simulink library "dit"  (Simulink 8.1)
settings: Solver=ode1  StartTime=0.0  StopTime=Inf  FixedStep=0.001  RelTol=1e-3
PostLoadFcn:
  | , if any(exist('dsrtsu_mdlpostloadfcn', 'file') == [2, 3, 6]), try dsrtsu_mdlpostloadfcn('Execute', bdroot); catch fprintf('Error in PostLoadFcn (dsrtsu_mdlpostloadfcn) for model "%s":\n %s\n', bdroot, lasterr); end, end,
undefined symbols (not defined in the file or in its folder): KACC_TransDistIncMargin_m, KACC_TransitoryClearanceDec_m, KACC_TransitoryDesDistApproach_m, KACC_TransitoryDistIntrusion_m, KACC_TransitoryRelSpd_kph
libraries: hcu_lib x1
settings Model: DSRTSU_INTERNAL_RTI_VER=450  DSRTSU_INTERNAL_RTI_TYPE=rti1401  RTICANMMDATA=struct('GeneralSetupData',struct('modelroot','D:\ELN150201_TAIWAN\trunk\AdasDragon\software\sw_development\arch\app\acc','generalsettings',struct('filesettings',struct('destfolder',struct('Name','RTICANMM_FILES','Check',1),'buildfolder',struct('Name','.','Check',1),'AbsDestfolder',struct('Name','D:\ELN150201_TAIWAN\trunk\AdasDragon\software\sw_development\arch\app\acc\RTICANMM_FILES'),'AbsBuildfolder',struct('Name','D:\ELN150201_TAIWAN\trunk\AdasDragon\software\sw_development\arch\app\acc'))),'options',struct('addpaths',1,'rmpaths',1,'addtrcexclusion',logical(1),'cannavigator',struct('checkmonitoring',0),'show_usrtrc',0,'use_usrtrc',0),'advanced',struct('options',[1 1 1 1 1 1 1 1 1 1 1 1 1 1 1 1 1 1 1 1 1 1 1 1 1 1 1 1 1 1 1 1 1 1 1 1 1 1 1 1 1 1 1 1 1 1 1 1 1 1 1 1 1 1 1 1 1 1 1 1 1 1 1 1 1 1 1 1 1 1 1 1 1 1 1 1 1 1 1 1 1 1 1 1 1 1 1 1 1 1 1 1 1 1 1 1 1 1 1 1]),'MPSetup',{{}},'modelname','dit','block','dit'))  DSRTSU_INTERNAL_RTIFPGA=40  Creator=AT015411  LastModifiedBy=AT015555

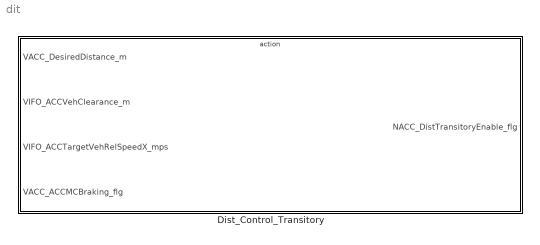
== system dit ==
  Dist_Control_Transitory : Subsystem  TreatAsAtomicUnit=on

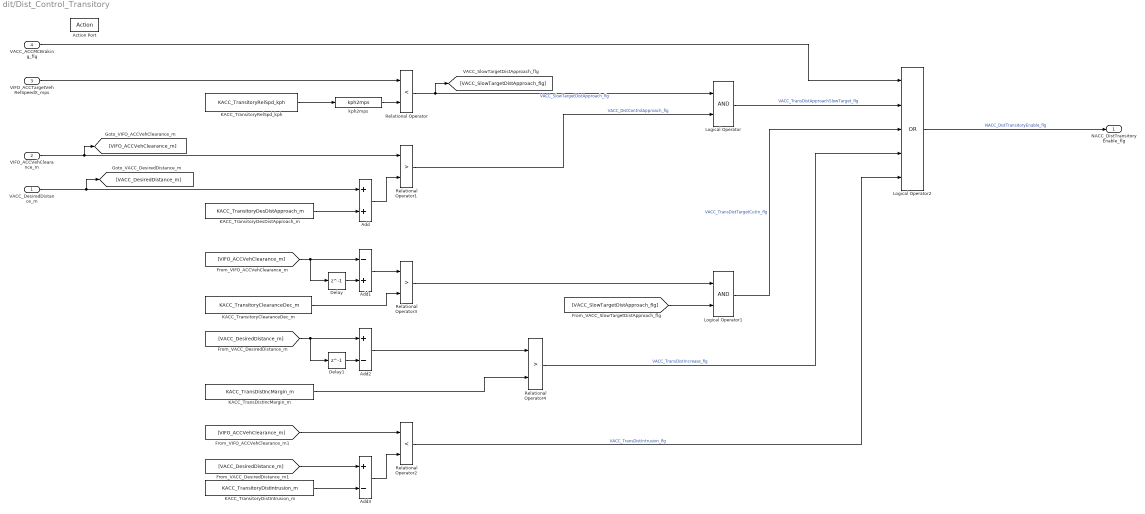
== system dit/Dist_Control_Transitory ==
  VACC_DesiredDistance_m : Inport
  VIFO_ACCVehClearance_m : Inport  Port=2
  VIFO_ACCTargetVehRelSpeedX_mps : Inport  Port=3
  VACC_ACCMCBraking_flg : Inport  Port=4
  Action Port : ActionPort
  Add : Sum
  Add1 : Sum  Inputs=-+
  Add2 : Sum  Inputs=+-
  Add3 : Sum  Inputs=+-
  Delay : Delay  DelayLength=1  InitialCondition=0
  Delay1 : Delay  DelayLength=1  InitialCondition=0
  KACC_TransDistIncMargin_m : Constant  Value=KACC_TransDistIncMargin_m
  KACC_TransitoryClearanceDec_m : Constant  Value=KACC_TransitoryClearanceDec_m
  KACC_TransitoryDesDistApproach_m : Constant  Value=KACC_TransitoryDesDistApproach_m
  KACC_TransitoryDistIntrusion_m : Constant  Value=KACC_TransitoryDistIntrusion_m
  KACC_TransitoryRelSpd_kph : Constant  Value=KACC_TransitoryRelSpd_kph
  Logical Operator : Logic  AllPortsSameDT=off  OutDataTypeStr=boolean
  Logical Operator1 : Logic  AllPortsSameDT=off  OutDataTypeStr=boolean
  Logical Operator2 : Logic  Operator=OR  Inputs=5  AllPortsSameDT=off  OutDataTypeStr=boolean
  Relational Operator : RelationalOperator  Operator=<  OutDataTypeStr=boolean
  Relational Operator1 : RelationalOperator  Operator=>  OutDataTypeStr=boolean
  Relational Operator2 : RelationalOperator  Operator=<  OutDataTypeStr=boolean
  Relational Operator3 : RelationalOperator  Operator=>  OutDataTypeStr=boolean
  Relational Operator4 : RelationalOperator  Operator=>  OutDataTypeStr=boolean
  kph2mps : hcu_lib/kph2mps
  NACC_DistTransitoryEnable_flg : Outport
  wires:
  VIFO_ACCTargetVehRelSpeedX_mps/1 -> Relational Operator/1
  KACC_TransitoryRelSpd_kph/1 -> kph2mps/1
  kph2mps/1 -> Relational Operator/2
  VIFO_ACCVehClearance_m/1 -> [VIFO_ACCVehClearance_m], Relational Operator1/1
  VACC_DesiredDistance_m/1 -> [VACC_DesiredDistance_m], Add/1
  KACC_TransitoryDesDistApproach_m/1 -> Add/2
  Add/1 -> Relational Operator1/2
  Relational Operator/1 -> Logical Operator/1, [VACC_SlowTargetDistApproach_flg]  "VACC_SlowTargetDistApproach_flg"
  Relational Operator1/1 -> Logical Operator/2  "VACC_DistControlApproach_flg"
  [VIFO_ACCVehClearance_m] -> Delay/1, Add1/1
  Delay/1 -> Add1/2
  Add1/1 -> Relational Operator3/1
  Relational Operator3/1 -> Logical Operator1/1
  [VACC_SlowTargetDistApproach_flg] -> Logical Operator1/2
  [VACC_DesiredDistance_m] -> Add2/1, Delay1/1
  Delay1/1 -> Add2/2
  Add2/1 -> Relational Operator4/1
  Relational Operator4/1 -> Logical Operator2/4  "VACC_TransDistIncrease_flg"
  [VIFO_ACCVehClearance_m] -> Relational Operator2/1
  [VACC_DesiredDistance_m] -> Add3/1
  KACC_TransitoryDistIntrusion_m/1 -> Add3/2
  Add3/1 -> Relational Operator2/2
  Logical Operator/1 -> Logical Operator2/2  "VACC_TransDistApproachSlowTarget_flg"
  VACC_ACCMCBraking_flg/1 -> Logical Operator2/1
  Logical Operator1/1 -> Logical Operator2/3  "VACC_TransDistTargetCutIn_flg"
  Relational Operator2/1 -> Logical Operator2/5  "VACC_TransDistIntrusion_flg"
  Logical Operator2/1 -> NACC_DistTransitoryEnable_flg/1  "NACC_DistTransitoryEnable_flg"
  KACC_TransitoryClearanceDec_m/1 -> Relational Operator3/2
  KACC_TransDistIncMargin_m/1 -> Relational Operator4/2
